simulink model "TST_PTSSE_SetData"  (R2016b)
settings: Solver=FixedStepDiscrete  StartTime=0.0  StopTime=simTime  FixedStep=sampleTime  RelTol=1e-3
values from neighbouring files (symbols this model uses):
  testCase = 1    [initTST_PTSSE_SetData_001.m]
libraries: simulink x2
settings Model: Creator=WF305  LastModifiedBy=WF305
settings DebuggingCC: SignalRangeChecking=error

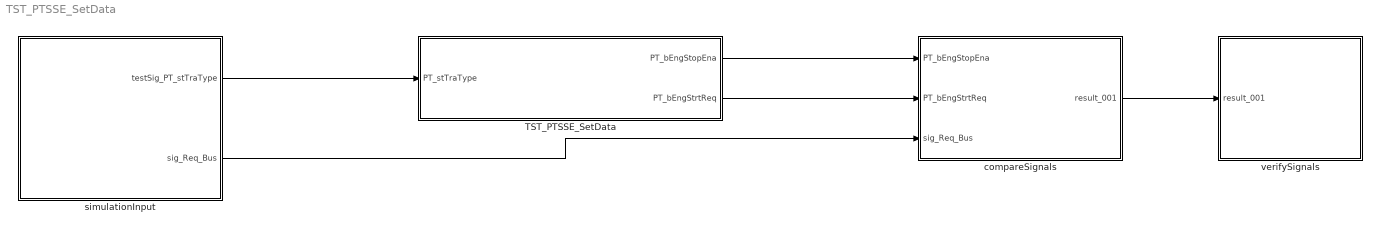
== system TST_PTSSE_SetData ==
  TST_PTSSE_SetData : Subsystem
  compareSignals : Subsystem
  simulationInput : Subsystem
  verifySignals : Subsystem
  wires:
  simulationInput/1(testSig_PT_stTraType) -> TST_PTSSE_SetData/1(PT_stTraType)
  TST_PTSSE_SetData/1(PT_bEngStopEna) -> compareSignals/1(PT_bEngStopEna)
  TST_PTSSE_SetData/2(PT_bEngStrtReq) -> compareSignals/2(PT_bEngStrtReq)
  simulationInput/2(sig_Req_Bus) -> compareSignals/3(sig_Req_Bus)
  compareSignals/1(result_001) -> verifySignals/1(result_001)

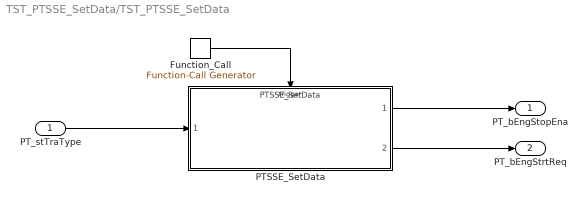
== system TST_PTSSE_SetData/TST_PTSSE_SetData ==
  PT_stTraType : Inport
  Function_Call : simulink/Ports & Subsystems/Function-Call Generator  sample_time=sampleTime  numberOfIterations=1
  PTSSE_SetData : ModelReference  ModelNameDialog=PTSSE_SetData  ModelReferenceVersion=1.2  TriggerPortName=function  TriggerPortTriggerType=function-call  TriggerPortStatesWhenEnabling=held
  PT_bEngStopEna : Outport
  PT_bEngStrtReq : Outport  Port=2
  wires:
  Function_Call/1 -> PTSSE_SetData/Trigger
  PT_stTraType/1 -> PTSSE_SetData/1
  PTSSE_SetData/1 -> PT_bEngStopEna/1
  PTSSE_SetData/2 -> PT_bEngStrtReq/1

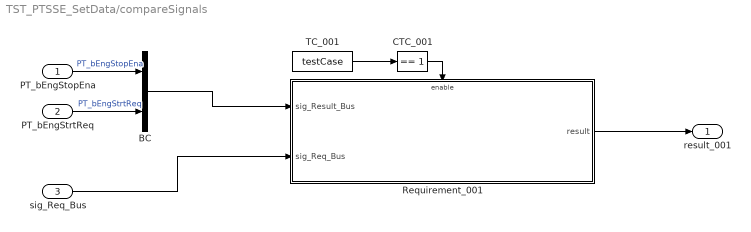
== system TST_PTSSE_SetData/compareSignals ==
  PT_bEngStopEna : Inport
  PT_bEngStrtReq : Inport  Port=2
  sig_Req_Bus : Inport  Port=3
  BC : BusCreator  Inputs=2
  CTC_001 : simulink/Logic and Bit Operations/Compare To Constant  relop===  const=1  OutDataTypeStr=boolean
  Requirement_001 : Subsystem
  TC_001 : Constant  Value=testCase
  result_001 : Outport
  wires:
  PT_bEngStopEna/1 -> BC/1  "PT_bEngStopEna"
  PT_bEngStrtReq/1 -> BC/2  "PT_bEngStrtReq"
  TC_001/1 -> CTC_001/1
  CTC_001/1 -> Requirement_001/Enable
  sig_Req_Bus/1 -> Requirement_001/2(sig_Req_Bus)
  BC/1 -> Requirement_001/1(sig_Result_Bus)
  Requirement_001/1(result) -> result_001/1

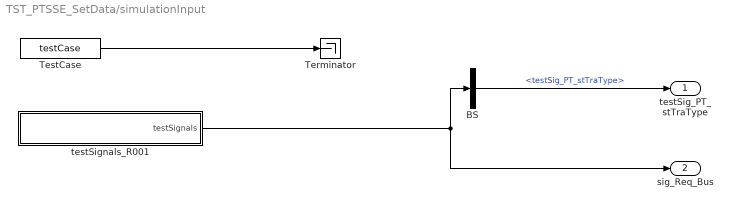
== system TST_PTSSE_SetData/simulationInput ==
  BS : BusSelector  OutputSignals=testSig_PT_stTraType
  Terminator : Terminator
  TestCase : Constant  Value=testCase
  testSignals_R001 : Subsystem
  testSig_PT_stTraType : Outport
  sig_Req_Bus : Outport  Port=2
  wires:
  BS/1 -> testSig_PT_stTraType/1  "<testSig_PT_stTraType>"
  testSignals_R001/1(testSignals) -> BS/1, sig_Req_Bus/1
  TestCase/1 -> Terminator/1

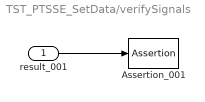
== system TST_PTSSE_SetData/verifySignals ==
  result_001 : Inport
  Assertion_001 : Assertion
  wires:
  result_001/1 -> Assertion_001/1

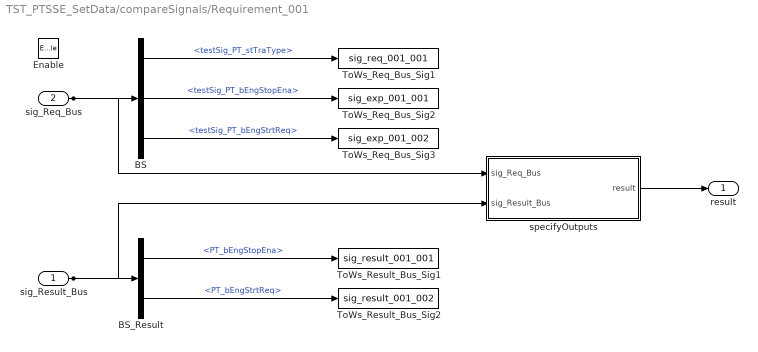
== system TST_PTSSE_SetData/compareSignals/Requirement_001 ==
  sig_Result_Bus : Inport
  sig_Req_Bus : Inport  Port=2
  Enable : EnablePort
  BS : BusSelector  OutputSignals=testSig_PT_stTraType,testSig_PT_bEngStopEna,testSig_PT_bEngStrtReq
  BS_Result : BusSelector  OutputSignals=PT_bEngStopEna,PT_bEngStrtReq
  ToWs_Req_Bus_Sig1 : ToWorkspace  VariableName=sig_req_001_001  SaveFormat=Structure With Time
  ToWs_Req_Bus_Sig2 : ToWorkspace  VariableName=sig_exp_001_001  SaveFormat=Structure With Time
  ToWs_Req_Bus_Sig3 : ToWorkspace  VariableName=sig_exp_001_002  SaveFormat=Structure With Time
  ToWs_Result_Bus_Sig1 : ToWorkspace  VariableName=sig_result_001_001  SaveFormat=Structure With Time
  ToWs_Result_Bus_Sig2 : ToWorkspace  VariableName=sig_result_001_002  SaveFormat=Structure With Time
  specifyOutputs : Subsystem
  result : Outport
  wires:
  sig_Req_Bus/1 -> BS/1, specifyOutputs/1(sig_Req_Bus)
  BS/1 -> ToWs_Req_Bus_Sig1/1  "<testSig_PT_stTraType>"
  BS/2 -> ToWs_Req_Bus_Sig2/1  "<testSig_PT_bEngStopEna>"
  BS/3 -> ToWs_Req_Bus_Sig3/1  "<testSig_PT_bEngStrtReq>"
  sig_Result_Bus/1 -> BS_Result/1, specifyOutputs/2(sig_Result_Bus)
  BS_Result/1 -> ToWs_Result_Bus_Sig1/1  "<PT_bEngStopEna>"
  BS_Result/2 -> ToWs_Result_Bus_Sig2/1  "<PT_bEngStrtReq>"
  specifyOutputs/1(result) -> result/1

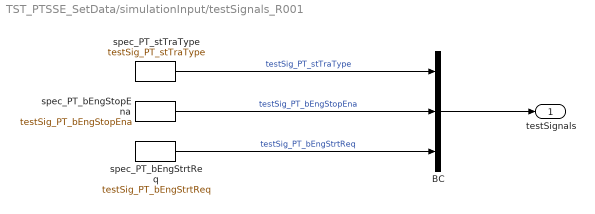
== system TST_PTSSE_SetData/simulationInput/testSignals_R001 ==
  BC : BusCreator  Inputs=3
  spec_PT_bEngStopEna : FromWorkspace  VariableName=testSig_PT_bEngStopEna  Interpolate=off  OutputAfterFinalValue=Holding final value
  spec_PT_bEngStrtReq : FromWorkspace  VariableName=testSig_PT_bEngStrtReq  Interpolate=off  OutputAfterFinalValue=Holding final value
  spec_PT_stTraType : FromWorkspace  VariableName=testSig_PT_stTraType  Interpolate=off  OutputAfterFinalValue=Holding final value
  testSignals : Outport
  wires:
  BC/1 -> testSignals/1
  spec_PT_stTraType/1 -> BC/1  "testSig_PT_stTraType"
  spec_PT_bEngStopEna/1 -> BC/2  "testSig_PT_bEngStopEna"
  spec_PT_bEngStrtReq/1 -> BC/3  "testSig_PT_bEngStrtReq"

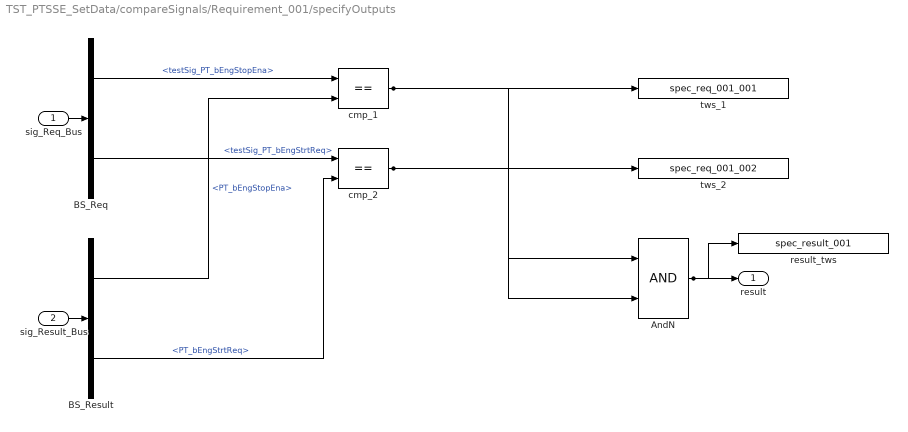
== system TST_PTSSE_SetData/compareSignals/Requirement_001/specifyOutputs ==
  sig_Req_Bus : Inport
  sig_Result_Bus : Inport  Port=2
  AndN : Logic
  BS_Req : BusSelector  OutputSignals=testSig_PT_bEngStopEna,testSig_PT_bEngStrtReq
  BS_Result : BusSelector  OutputSignals=PT_bEngStopEna,PT_bEngStrtReq
  cmp_1 : RelationalOperator  Operator===  RndMeth=Nearest  InputSameDT=on
  cmp_2 : RelationalOperator  Operator===  RndMeth=Nearest  InputSameDT=on
  result_tws : ToWorkspace  VariableName=spec_result_001
  tws_1 : ToWorkspace  VariableName=spec_req_001_001
  tws_2 : ToWorkspace  VariableName=spec_req_001_002
  result : Outport
  wires:
  sig_Req_Bus/1 -> BS_Req/1
  sig_Result_Bus/1 -> BS_Result/1
  AndN/1 -> result/1, result_tws/1
  BS_Req/1 -> cmp_1/1  "<testSig_PT_bEngStopEna>"
  BS_Result/1 -> cmp_1/2  "<PT_bEngStopEna>"
  cmp_1/1 -> tws_1/1, AndN/1
  BS_Req/2 -> cmp_2/1  "<testSig_PT_bEngStrtReq>"
  BS_Result/2 -> cmp_2/2  "<PT_bEngStrtReq>"
  cmp_2/1 -> tws_2/1, AndN/2
